simulink model "proj"  (Simulink 5.0)
settings: Solver=ode1  SolverMode=SingleTasking  StartTime=0.0  StopTime=70.0  FixedStep=0.001  RelTol=1e-3
InitFcn:
  | init_para
undefined symbols (not defined in the file): a, dzcv, fc, fp, fs, g, j, l, M, mi, xc, yc
settings Model: LastModifiedBy=AD  BooleanDataType=off

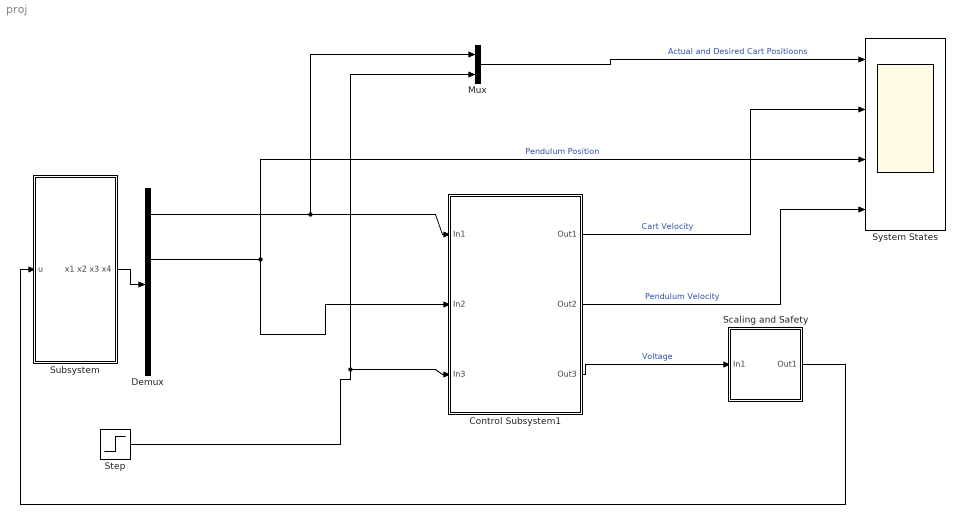
== system proj ==
  Control Subsystem1 : Subsystem
  Demux : Demux
  Mux : Mux  Inputs=2
  Scaling and Safety : Subsystem
  Step : Step  SampleTime=0
  Subsystem : Subsystem
  System States : Scope  NumInputPorts=4
      settings: TimeRange=70  YMin=-0.1~-0.15~-3.18~-0.35  YMax=0.15~0.125~-3.125~0.3  Decimation=0.1  SampleInput=on  SampleTime=0.01
  wires:
  Scaling and Safety/1(Out1) -> Subsystem/1(u)
  Mux/1 -> System States/1  "Actual and Desired Cart Positioons"
  Control Subsystem1/1(Out1) -> System States/2  "Cart Velocity"
  Control Subsystem1/2(Out2) -> System States/4  "Pendulum Velocity"
  Control Subsystem1/3(Out3) -> Scaling and Safety/1(In1)  "Voltage"
  Subsystem/1(x1 x2 x3 x4) -> Demux/1
  Demux/1 -> Mux/1, Control Subsystem1/1(In1)
  Demux/2 -> System States/3, Control Subsystem1/2(In2)  "Pendulum Position"
  Step/1 -> Mux/2, Control Subsystem1/3(In3)

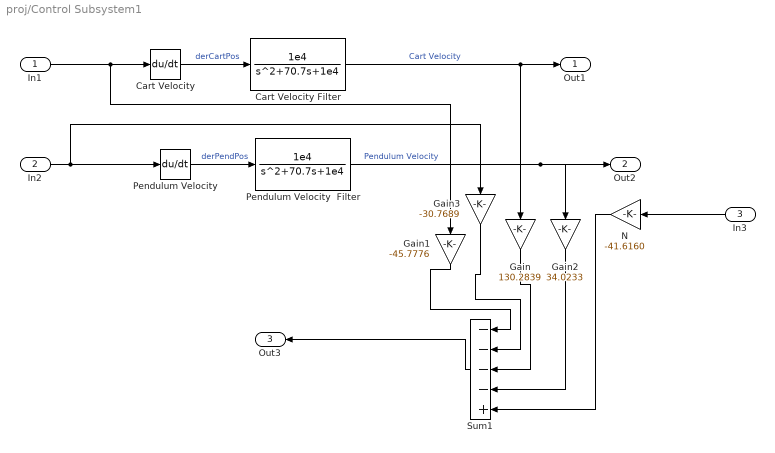
== system proj/Control Subsystem1 ==
  In1 : Inport
  In2 : Inport  Port=2
  In3 : Inport  Orientation=left  Port=3
  Cart Velocity : Derivative
  Cart Velocity Filter : TransferFcn  Numerator=[1e4]  Denominator=[1 70.7 1e4]
  Gain : Gain  Orientation=down  Gain=130.2839  SaturateOnIntegerOverflow=on
  Gain1 : Gain  Orientation=down  Gain=-45.7776  SaturateOnIntegerOverflow=on
  Gain2 : Gain  Orientation=down  Gain=34.0233  SaturateOnIntegerOverflow=on
  Gain3 : Gain  Orientation=down  Gain=-30.7689  SaturateOnIntegerOverflow=on
  N : Gain  Orientation=left  Gain=-41.6160  SaturateOnIntegerOverflow=on
  Pendulum Velocity : Derivative
  Pendulum Velocity  Filter : TransferFcn  Numerator=[1e4]  Denominator=[1 70.7 1e4]
  Sum1 : Sum  Orientation=left  Inputs=----+  SaturateOnIntegerOverflow=on  InputSameDT=on
  Out1 : Outport
  Out2 : Outport  Port=2
  Out3 : Outport  Orientation=left  Port=3
  wires:
  N/1 -> Sum1/5
  Sum1/1 -> Out3/1
  Gain2/1 -> Sum1/4
  Gain3/1 -> Sum1/2
  Gain/1 -> Sum1/3
  Gain1/1 -> Sum1/1
  In2/1 -> Gain3/1, Pendulum Velocity/1
  In1/1 -> Gain1/1, Cart Velocity/1
  Pendulum Velocity  Filter/1 -> Gain2/1, Out2/1  "Pendulum Velocity"
  Cart Velocity Filter/1 -> Gain/1, Out1/1  "Cart Velocity"
  Pendulum Velocity/1 -> Pendulum Velocity  Filter/1  "derPendPos"
  Cart Velocity/1 -> Cart Velocity Filter/1  "derCartPos"
  In3/1 -> N/1

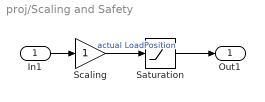
== system proj/Scaling and Safety ==
  In1 : Inport
  Saturation : Saturate  UpperLimit=2.5  LowerLimit=-2.5
  Scaling : Gain  SaturateOnIntegerOverflow=on
  Out1 : Outport
  wires:
  Scaling/1 -> Saturation/1  "actual LoadPosition"
  In1/1 -> Scaling/1
  Saturation/1 -> Out1/1

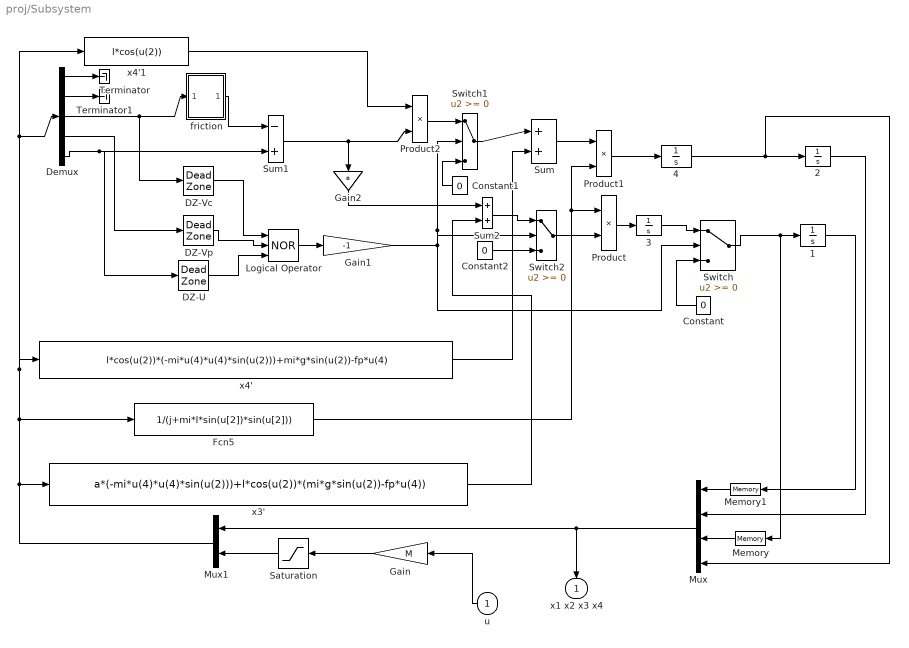
== system proj/Subsystem ==
  u : Inport  Orientation=left
  {1..4} (4 alike) : Integrator
  Constant : Constant  Orientation=left  Value=0
  Constant1 : Constant  Orientation=left  Value=0
  Constant2 : Constant  Value=0
  DZ-U : DeadZone  LowerValue=-1.37918  UpperValue=1.37918  SaturateOnIntegerOverflow=on
  DZ-Vc : DeadZone  LowerValue=-0.00793711  UpperValue=0.00793711  SaturateOnIntegerOverflow=on
  DZ-Vp : DeadZone  LowerValue=-3.37476  UpperValue=3.37476  SaturateOnIntegerOverflow=on
  Demux : Demux  Outputs=5
  Fcn5 : Fcn  Expr=1/(j+mi*l*sin(u[2])*sin(u[2]))
  Gain : Gain  Orientation=left  Gain=M  SaturateOnIntegerOverflow=on
  Gain1 : Gain  Gain=-1  SaturateOnIntegerOverflow=on
  Gain2 : Gain  Orientation=down  Gain=a  SaturateOnIntegerOverflow=on
  Logical Operator : Logic  Operator=NOR  Inputs=3  AllPortsSameDT=off
  Memory : Memory  Orientation=left
  Memory1 : Memory  Orientation=left
  Mux : Mux  Orientation=left
  Mux1 : Mux  Orientation=left  Inputs=2
  Product : Product  SaturateOnIntegerOverflow=on
  Product1 : Product  SaturateOnIntegerOverflow=on
  Product2 : Product  SaturateOnIntegerOverflow=on
  Saturation : Saturate  Orientation=left  UpperLimit=5  LowerLimit=-5
  Sum : Sum  Inputs=|++  SaturateOnIntegerOverflow=on
  Sum1 : Sum  Inputs=-+  SaturateOnIntegerOverflow=on
  Sum2 : Sum  SaturateOnIntegerOverflow=on
  Switch : Switch  SaturateOnIntegerOverflow=on
  Switch1 : Switch  SaturateOnIntegerOverflow=on
  Switch2 : Switch  SaturateOnIntegerOverflow=on
  Terminator : Terminator
  Terminator1 : Terminator
  friction : Subsystem
  x3' : Fcn  Expr=a*(-mi*u(4)*u(4)*sin(u(2)))+l*cos(u(2))*(mi*g*sin(u(2))-fp*u(4))
  x4' : Fcn  Expr=l*cos(u(2))*(-mi*u(4)*u(4)*sin(u(2)))+mi*g*sin(u(2))-fp*u(4)
  x4'1 : Fcn  Expr=l*cos(u(2))
  x1 x2 x3 x4 : Outport  Orientation=down
  wires:
  Gain1/1 -> Switch2/2, Switch1/2, Switch/2
  Sum1/1 -> Gain2/1, Product2/2
  Demux/5 -> Sum1/2, DZ-U/1
  4/1 -> Mux/4, 2/1
  friction/1(out-1) -> Sum1/1
  Demux/2 -> Terminator1/1
  Demux/1 -> Terminator/1
  Gain2/1 -> Sum2/1
  x3'/1 -> Sum2/2
  Sum2/1 -> Switch2/1
  Memory1/1 -> Mux/1
  Constant2/1 -> Switch2/3
  Switch2/1 -> Product/2
  Logical Operator/1 -> Gain1/1
  DZ-U/1 -> Logical Operator/3
  DZ-Vp/1 -> Logical Operator/2
  DZ-Vc/1 -> Logical Operator/1
  Sum/1 -> Product1/1
  Memory/1 -> Mux/3
  1/1 -> Memory1/1
  2/1 -> Mux/2
  3/1 -> Switch/1
  Switch/1 -> Memory/1, 1/1
  Saturation/1 -> Mux1/2
  Mux/1 -> x1 x2 x3 x4/1, Mux1/1
  Mux1/1 -> Demux/1, x4'1/1, x4'/1, Fcn5/1, x3'/1
  Gain/1 -> Saturation/1
  Product/1 -> 3/1
  Product1/1 -> 4/1
  Fcn5/1 -> Product/1, Product1/2
  x4'/1 -> Sum/2
  Switch1/1 -> Sum/1
  Product2/1 -> Switch1/1
  x4'1/1 -> Product2/1
  Constant/1 -> Switch/3
  Constant1/1 -> Switch1/3
  Demux/4 -> DZ-Vp/1
  Demux/3 -> friction/1(In1), DZ-Vc/1
  u/1 -> Gain/1

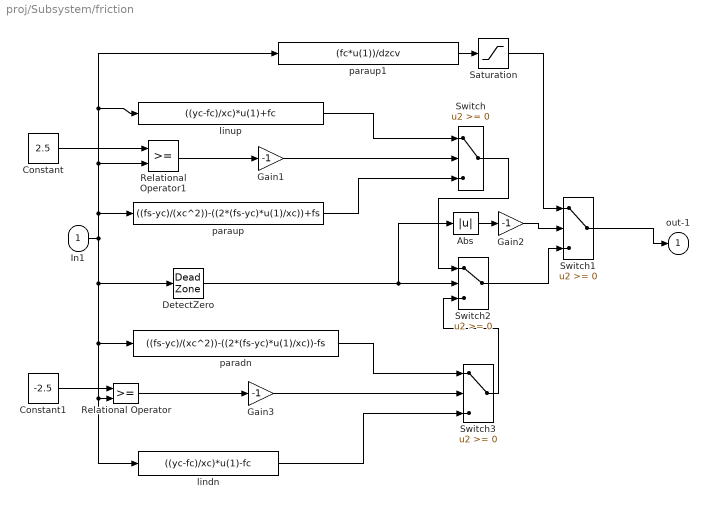
== system proj/Subsystem/friction ==
  In1 : Inport
  Abs : Abs  SaturateOnIntegerOverflow=on
  Constant : Constant  Value=2.5
  Constant1 : Constant  Value=-2.5
  DetectZero : DeadZone  SaturateOnIntegerOverflow=on
  Gain1 : Gain  Gain=-1  SaturateOnIntegerOverflow=on
  Gain2 : Gain  Gain=-1  SaturateOnIntegerOverflow=on
  Gain3 : Gain  Gain=-1  SaturateOnIntegerOverflow=on
  Relational Operator : RelationalOperator
  Relational Operator1 : RelationalOperator
  Saturation : Saturate
  Switch{,1..3} (4 alike) : Switch  SaturateOnIntegerOverflow=on
  lindn : Fcn  Expr=((yc-fc)/xc)*u(1)-fc
  linup : Fcn  Expr=((yc-fc)/xc)*u(1)+fc
  paradn : Fcn  Expr=((fs-yc)/(xc^2))-((2*(fs-yc)*u(1)/xc))-fs
  paraup : Fcn  Expr=((fs-yc)/(xc^2))-((2*(fs-yc)*u(1)/xc))+fs
  paraup1 : Fcn  Expr=(fc*u(1))/dzcv
  out-1 : Outport
  wires:
  Gain3/1 -> Switch3/2
  Gain1/1 -> Switch/2
  paraup1/1 -> Saturation/1
  Relational Operator1/1 -> Gain1/1
  Constant1/1 -> Relational Operator/1
  Constant/1 -> Relational Operator1/1
  lindn/1 -> Switch3/3
  Relational Operator/1 -> Gain3/1
  paradn/1 -> Switch3/1
  Switch3/1 -> Switch2/3
  Switch2/1 -> Switch1/3
  Gain2/1 -> Switch1/2
  Abs/1 -> Gain2/1
  Switch/1 -> Switch2/1
  DetectZero/1 -> Abs/1, Switch2/2
  In1/1 -> paraup1/1, linup/1, Relational Operator1/2, paraup/1, DetectZero/1, lindn/1, Relational Operator/2, paradn/1
  paraup/1 -> Switch/3
  linup/1 -> Switch/1
  Saturation/1 -> Switch1/1
  Switch1/1 -> out-1/1
